simulink model "simulink"  (R2016a)
settings: Solver=VariableStepAuto  StartTime=0.0  StopTime=518400  RelTol=1e-3
values from neighbouring files (symbols this model uses):
  Ad = 0.606534330298    [sysd.mat]    (also in trock.m = sysdd.A)
  Bd = [-0.0242754206752 -0.00855612972972]    [sysd.mat]    (also in trock.m = sysdd.B(1:2))
  Cd = [0.128107607141 0.111213837289]    [sysd.mat]    (also in trock.m = sysdd.C)
  Dd = [-0.0321285947629  0.0590346867599; -0.035674975325  0.0556784277831]    [sysd.mat]    (also in trock.m = sysdd.D(:,1:2))
  Ed = sysdd.B(3:4)    [trock.m]
  Kd = sysdd.D(:,3:4)    [trock.m]
  Ts = 87.5440    (= 87.544)    [Initialization.m]    (also in MPC_test.m = 6.4385; sysd.mat = 6.4385; trock.m)
libraries: simulink x2
settings Model: Creator=Trojass  LastModifiedBy=Trojass

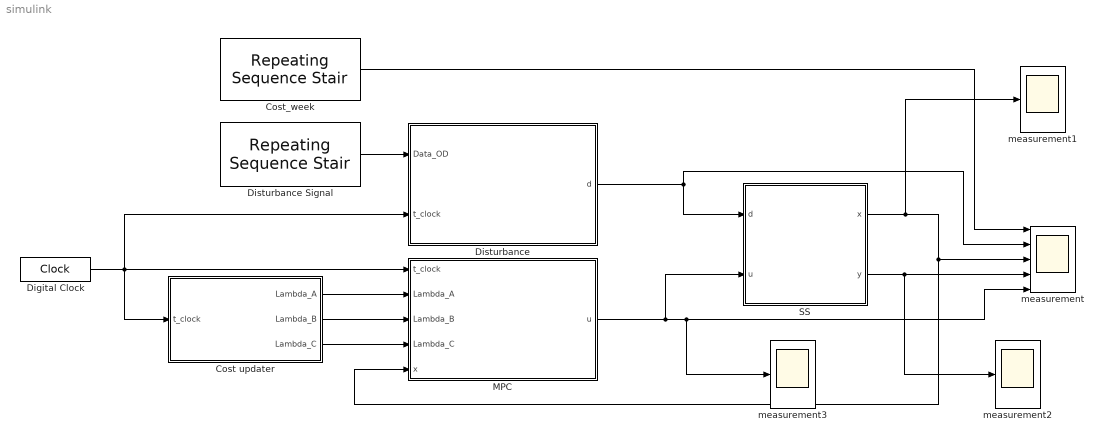
== system simulink ==
  Cost updater : Subsystem
  Cost_week : simulink/Sources/Repeating Sequence Stair  OutValues=data  tsamp=3600  OutMin=[]  OutMax=[]  OutDataTypeStr=double  OutputDataTypeScalingMode=double  OutDataType=fixdt(0,8)  ConRadixGroup=Best Precision: Vector-wise  OutScaling=2^-12
  Digital Clock : DigitalClock  SampleTime=Ts
  "Disturbance " : MATLAB Function  TreatAsAtomicUnit=on
  Disturbance Signal : simulink/Sources/Repeating Sequence Stair  OutValues=constant_dist  tsamp=3600  OutMin=[]  OutMax=[]  OutDataTypeStr=double  OutputDataTypeScalingMode=double  OutDataType=fixdt(0,8)  ConRadixGroup=Best Precision: Vector-wise  OutScaling=2^-12
  MPC : Subsystem
  SS : Subsystem
  measurement : Scope  NumInputPorts=5
  measurement1 : Scope
  measurement2 : Scope
  measurement3 : Scope
  wires:
  SS/2(y) -> measurement2/1, measurement/4
  SS/1(x) -> measurement1/1, measurement/3, MPC/5(x)
  Digital Clock/1 -> MPC/1(t_clock), "Disturbance "/2(t_clock), Cost updater/1(t_clock)
  "Disturbance "/1(d) -> measurement/2, SS/1(d)
  Disturbance Signal/1 -> "Disturbance "/1(Data_OD)
  MPC/1(u) -> measurement3/1, measurement/5, SS/2(u)
  Cost updater/1(Lambda_A) -> MPC/2(Lambda_A)
  Cost updater/2(Lambda_B) -> MPC/3(Lambda_B)
  Cost updater/3(Lambda_C) -> MPC/4(Lambda_C)
  Cost_week/1 -> measurement/1

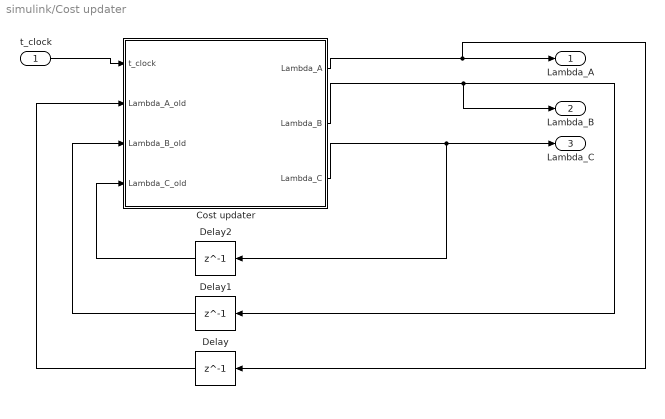
== system simulink/Cost updater ==
  t_clock : Inport
  "Cost updater " : MATLAB Function  TreatAsAtomicUnit=on
  Delay : Delay  DelayLength=1  InitialCondition=0  SampleTime=Ts
  Delay1 : Delay  DelayLength=1  InitialCondition=0  SampleTime=Ts
  Delay2 : Delay  DelayLength=1  InitialCondition=0  SampleTime=Ts
  Lambda_A : Outport
  Lambda_B : Outport  Port=2
  Lambda_C : Outport  Port=3
  wires:
  "Cost updater "/1(Lambda_A) -> Delay/1, Lambda_A/1
  Delay2/1 -> "Cost updater "/4(Lambda_C_old)
  "Cost updater "/2(Lambda_B) -> Lambda_B/1, Delay1/1
  Delay/1 -> "Cost updater "/2(Lambda_A_old)
  Delay1/1 -> "Cost updater "/3(Lambda_B_old)
  "Cost updater "/3(Lambda_C) -> Lambda_C/1, Delay2/1
  t_clock/1 -> "Cost updater "/1(t_clock)

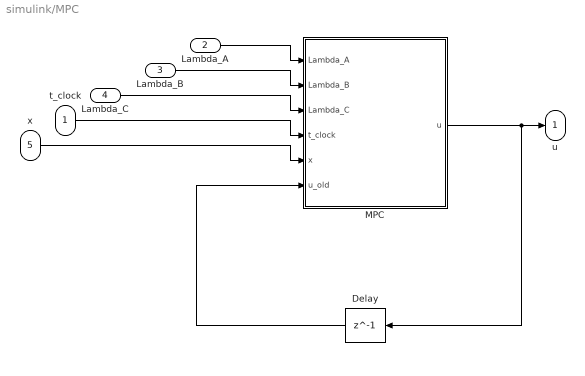
== system simulink/MPC ==
  t_clock : Inport
  Lambda_A : Inport  Port=2
  Lambda_B : Inport  Port=3
  Lambda_C : Inport  Port=4
  x : Inport  Port=5
  Delay : Delay  DelayLength=1  InitialCondition=0  SampleTime=Ts
  MPC : MATLAB Function  TreatAsAtomicUnit=on
  u : Outport
  wires:
  x/1 -> MPC/5(x)
  t_clock/1 -> MPC/4(t_clock)
  Delay/1 -> MPC/6(u_old)
  MPC/1(u) -> Delay/1, u/1
  Lambda_B/1 -> MPC/2(Lambda_B)
  Lambda_C/1 -> MPC/3(Lambda_C)
  Lambda_A/1 -> MPC/1(Lambda_A)

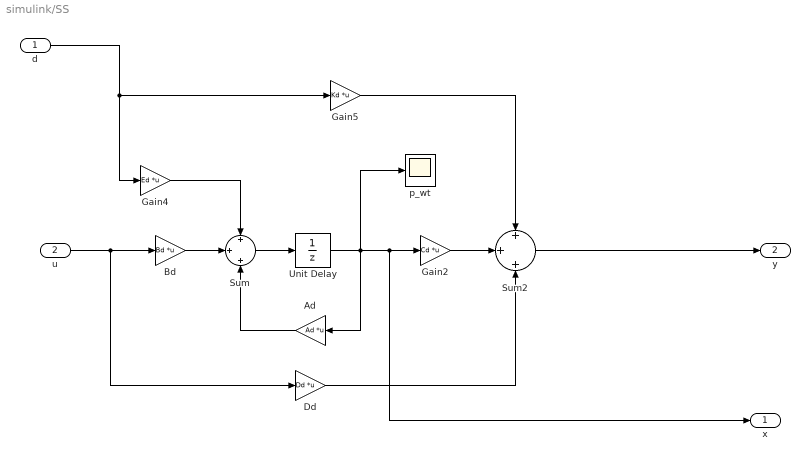
== system simulink/SS ==
  d : Inport
  u : Inport  Port=2
  Ad : Gain  Gain=Ad  Multiplication=Matrix(K*u)
      mask Display:
      | %color('cyan')
      | color('magenta')
      | disp('{\bf\fontsize{14}Ad}', 'texmode','on');
      | %disp('Ad')
  Bd : Gain  Gain=Bd  Multiplication=Matrix(K*u)
      mask Display:
      | %color('cyan')
      | color('magenta')
      | disp('{\bf\fontsize{14}Bd}', 'texmode','on');
      | %disp('Bd')
  Dd : Gain  Gain=Dd  Multiplication=Matrix(K*u)
      mask Display:
      | %color('cyan')
      | color('magenta')
      | disp('{\bf\fontsize{14}Dd}', 'texmode','on');
      | %disp('Dd')
  Gain2 : Gain  Gain=Cd  Multiplication=Matrix(K*u)
      mask Display:
      | %color('cyan')
      | color('magenta')
      | disp('{\bf\fontsize{14}Cd}', 'texmode','on');
      | %disp('Cd')
  Gain4 : Gain  Gain=Ed  Multiplication=Matrix(K*u)
      mask Display:
      | %color('cyan')
      | color('magenta')
      | disp('{\bf\fontsize{14}Ed}', 'texmode','on');
      | %disp('Ed')
  Gain5 : Gain  Gain=Kd  Multiplication=Matrix(K*u)
      mask Display:
      | %color('cyan')
      | color('magenta')
      | disp('{\bf\fontsize{14}Kd}', 'texmode','on');
      | %disp('Kd')
  Sum : Sum  Inputs=+|+|+
  Sum2 : Sum  Inputs=+|+|+
  Unit Delay : UnitDelay  InitialCondition=0.005  SampleTime=Ts
  p_wt : Scope
  x : Outport
  y : Outport  Port=2
  wires:
  Sum2/1 -> y/1
  Sum/1 -> Unit Delay/1
  Bd/1 -> Sum/2
  Ad/1 -> Sum/3
  Unit Delay/1 -> p_wt/1, x/1, Gain2/1, Ad/1
  u/1 -> Dd/1, Bd/1
  d/1 -> Gain4/1, Gain5/1
  Gain4/1 -> Sum/1
  Gain2/1 -> Sum2/2
  Dd/1 -> Sum2/3
  Gain5/1 -> Sum2/1

== matlab function simulink/Disturbance  ==
  data: Data_OD input; t_clock input; d output
function d   = fcn(Data_OD,t_clock)

% d_intt = load('Disturbance_Plot.mat');
% 
% d_int =[d_intt.Data_OD d_intt.Data_OD];
d_intt = load('constant_dist.mat');

d_int =[d_intt.constant_dist d_intt.constant_dist];


t_h = 1+floor(t_clock/3600);
if t_h / 24 ~= floor(t_h/24)
  t_int  = t_h - floor(t_h/24)*24;
else
  t_int = 24;
end

d = d_int(t_int,:)';

== matlab function simulink/MPC/MPC ==
  data: Lambda_A input; Lambda_B input; Lambda_C input; t_clock input; x input; u_old input; u output
function u  = fcn(Lambda_A, Lambda_B, Lambda_C,t_clock,x,u_old)
coder.extrinsic('optimoptions');
coder.extrinsic('fmincon');
coder.extrinsic('QP_func');
coder.extrinsic('quadprog');


%Time
Ts = 6.438500000000000;
t_h = 1+floor(t_clock/3600);
t_h_2 = 1+floor((t_clock-Ts)/3600);

if t_h ~= t_h_2
    %Define sizes
    u_hp = zeros(48,1);
    u_hp1 = zeros(24,1);
    u_hp2 = zeros(24,1);

    %Load system matrices
    data = load('data.mat');
    data = data.data;
    Gamma = load('Gamma.mat');
    Gamma = Gamma.Gamma;
    Omega = load('Omega.mat');
    Omega = Omega.Omega;
    Phi = load('Phi.mat');
    Phi = Phi.Phi;
    Pi = load('Pi.mat');
    Pi = Pi.Pi;
    Psi = load('Psi.mat');
    Psi = Psi.Psi;
    Theta = load('Theta.mat');
    Theta = Theta.Theta;
    %Load Disturbance
    constant_dist = load('constant_dist.mat');
    Data_OD = constant_dist.constant_dist;
    t_1 = 0:3600:3600*(length(Data_OD)-1);


    delta_p_0 = x;      %small-signal initial WT pressure measurement

    %d_hp = 0.025*90*ones(48,1);      % Small signal deviation of the Valves OD
    d_hp = [Data_OD(1,:); Data_OD(1,:);
            Data_OD(2,:); Data_OD(2,:);
            Data_OD(3,:); Data_OD(3,:);
            Data_OD(4,:); Data_OD(4,:);
            Data_OD(5,:); Data_OD(5,:);
            Data_OD(6,:); Data_OD(6,:);
            Data_OD(7,:); Data_OD(7,:);
            Data_OD(8,:); Data_OD(8,:);
            Data_OD(9,:); Data_OD(9,:);
            Data_OD(10,:); Data_OD(10,:);
            Data_OD(11,:); Data_OD(11,:);
            Data_OD(12,:); Data_OD(12,:);
            Data_OD(13,:); Data_OD(13,:);
            Data_OD(14,:); Data_OD(14,:);
            Data_OD(15,:); Data_OD(15,:);
            Data_OD(16,:); Data_OD(16,:);
            Data_OD(17,:); Data_OD(17,:);
            Data_OD(18,:); Data_OD(18,:);
            Data_OD(19,:); Data_OD(19,:);
            Data_OD(20,:); Data_OD(20,:);
            Data_OD(21,:); Data_OD(21,:);
            Data_OD(22,:); Data_OD(22,:);
            Data_OD(23,:); Data_OD(23,:);
            Data_OD(24,:); Data_OD(24,:)
            ];

    U_bar = 0.2;
    U_bar_hp = U_bar*ones(48,1);      % Input pressure to ring pumps operating point
    q_bar_p_hp = 0.45*ones(48,1);    % Flow operating point of the ring pumps

    %%%%%%%%%%%%%%%%%% General QP %%%%%%%%%%%%%%%%%%
    % 0.5*x'R*x+f'*x
    %%%%%%%%%%%%%%%%%%%%%%%%%%%%%%%%%%%%%%%%%%%%%%%%%%%%%%%
    %%%%%%%%%%%%%%%%%%%%% Constraint %%%%%%%%%%%%%%%%%%%%%%
    %%%%%%%%%%%%%%%%%%%%%%%%%%%%%%%%%%%%%%%%%%%%%%%%%%%%%%%

    % Output constraint
    y_low =  0.08*ones(48,1);         % Full-signal upper and lower bounds 
    y_high = 0.18*ones(48,1);           

    % Pressure operating point of the PMA end-users
    y_bar = [0.1562; 0.0991 ;0.1562; 0.0991 ;0.1562; 0.0991 ;0.1562; 0.0991 ;0.1562; 0.0991 ;0.1562; 0.0991 ;
            0.1562; 0.0991 ;0.1562; 0.0991 ;0.1562; 0.0991 ;0.1562; 0.0991 ;0.1562; 0.0991 ;0.1562; 0.0991 ;
            0.1562; 0.0991 ;0.1562; 0.0991 ;0.1562; 0.0991 ;0.1562; 0.0991 ;0.1562; 0.0991 ;0.1562; 0.0991 ;
            0.1562; 0.0991 ;0.1562; 0.0991 ;0.1562; 0.0991 ;0.1562; 0.0991 ;0.1562; 0.0991 ;0.1562; 0.0991];    

    y1 = y_low - y_bar - Theta*Phi*delta_p_0-(Theta*Psi+Pi)*d_hp + 0.2;
    y2 = y_high - y_bar - Theta*Phi*delta_p_0-(Theta*Psi+Pi)*d_hp + 0.1;
    L_y = Theta*Gamma+Omega;

    % State constraint
    x_low = 0.055*ones(24,1);
    x_high = 0.16*ones(24,1);
    x_bar = 0.127*ones(24,1);

    delta_p_wt_1 = x_low -x_bar - Phi*delta_p_0 - Psi*d_hp + 0.2;
    delta_p_wt_2 = x_high-x_bar - Phi*delta_p_0 - Psi*d_hp + 0.1;
    %delta_p_wt_2(1,1) = 0.014;
    % input constraint 
    u_low = [-0.17; -0.15 ;-0.17; -0.15 ;-0.17; -0.15 ;-0.17; -0.15 ;-0.17; -0.15 ;-0.17; -0.15 ;
        -0.17; -0.15 ;-0.17; -0.15 ;-0.17; -0.15 ;-0.17; -0.15 ;-0.17; -0.15 ;-0.17; -0.15 ;
        -0.17; -0.15 ;-0.17; -0.15 ;-0.17; -0.15 ;-0.17; -0.15 ;-0.17; -0.15 ;-0.17; -0.15 ;
        -0.17; -0.15 ;-0.17; -0.15 ;-0.17; -0.15 ;-0.17; -0.15 ;-0.17; -0.15 ;-0.17; -0.15 ];    

    u_high = 0.75;

    %%%%%%%%%%%%%%%%%%%%%%%%%%%%%%%%%%%%%%%%%%%%%%%%%%%%%%%
    %%%%%%%%%%%%%%%%%% Setting up the QP %%%%%%%%%%%%%%%%%% 
    %%%%%%%%%%%%%%%%%%%%%%%%%%%%%%%%%%%%%%%%%%%%%%%%%%%%%%%

    R = 2*(Lambda_A + Lambda_C*Gamma); 

    R1=(R+R')/2;
    R2=(R-R')/2;
    f = (U_bar_hp'*(Lambda_A+Lambda_C*Gamma)+d_hp'*(Lambda_B+Lambda_C*Psi)'+delta_p_0*(Lambda_C*Phi)'+q_bar_p_hp');

    %CONSTRAINTS FOR Y AND X
    A = [-L_y; L_y; -Gamma; Gamma];
    b = [y1; y2; delta_p_wt_1; delta_p_wt_2];


    lb = u_low;
    ub = u_high*ones(48,1);

%     func = QP_func(R,f);

    options = optimoptions('quadprog','Algorithm','interior-point-convex');
    u_hp = quadprog(R,f,[],[],[],[],[lb],[ub],[],options);

    %%%

    u_hp1 = u_hp(1:2:length(u_hp));
    u_hp2 = u_hp(2:2:length(u_hp));
    
%     figure
%     subplot(2,1,1)
%     plot(u_hp1)
%     hold on
%     plot(u_hp2)
%     grid on
%     subplot(2,1,2)
%     plot(data(t_h:t_h+23,:))
%     grid on
    
    u = [u_hp1(1,:); u_hp2(1,:)] ;
    u_old = u;  
    else 
    u = u_old;
end

== matlab function simulink/Cost updater/Cost updater  ==
  data: t_clock input; Lambda_A output; Lambda_B output; Lambda_C output; Lambda_A_old input; Lambda_B_old input; Lambda_C_old input
function [Lambda_A,Lambda_B,Lambda_C] = fcn(t_clock,Lambda_A_old,Lambda_B_old,Lambda_C_old)
coder.extrinsic('cost_update');

data = load('data.mat');
data = data.data; %

%Time
Ts = 6.438500000000000;
t_h = 1+floor(t_clock/3600);
t_h_2 = 1+floor((t_clock-Ts)/3600);

if t_clock == Ts || t_h ~= t_h_2
    %Define size of matrices 
    Lambda_A = zeros(48,48);
    Lambda_B = zeros(48,48);
    Lambda_C = zeros(48,24);

    %Data 
    G_2 = load('G_2.mat');
    G_2 = G_2.G_2;
    B_1 = load('B_1.mat');
    B_1 = B_1.B_1;
    M_c = load('M_c.mat');
    M_c = M_c.M_c;
    N_c = load('N_c.mat');
    N_c = N_c.N_c;
    Q_c = load('Q_c.mat');
    Q_c = Q_c.Q_c;
    B_0 = load('B_0.mat');
    B_0 = B_0.B_0;

    %Define Lambda_A/B/C
    Hp = 24;
    Lambda_1 =  G_2 * B_1' * (M_c \ N_c);
    Lambda_2 = - G_2 * B_1' * (M_c \ Q_c);
    Lambda_3 = - G_2 * B_1' * (M_c \ B_0);

    [Lambda_A,Lambda_B,Lambda_C] = cost_update(data,Lambda_1,Lambda_2,Lambda_3,Hp,t_h);
    
     Lambda_A_old = Lambda_A;
     Lambda_B_old = Lambda_B;
     Lambda_C_old = Lambda_C;
else
 Lambda_A = zeros(48,48)+Lambda_A_old;
 Lambda_B = zeros(48,48)+Lambda_B_old;
 Lambda_C = zeros(48,24)+Lambda_C_old;
end
